simulink model "harness"  (R2024b)
settings: Solver=VariableStepAuto  StartTime=0.0  StopTime=100  FixedStep=1/100  RelTol=1e-3
InitFcn:
  | init_fn()
undefined symbols (not defined in the file): sigbuilder_block
libraries: simulink x9
settings Model: PacingRate=100  Creator=Jacopo Sini  LastModifiedBy=WxxGr
settings DataIOCC: ReturnWorkspaceOutputs=off  ReturnWorkspaceOutputsName=out1
settings OptimizationCC: ReuseModelBlockBuffer=off
settings DebuggingCC: ParameterPrecisionLossMsg=none  UnconnectedInputMsg=warning  UnconnectedOutputMsg=warning  UnconnectedLineMsg=warning
settings ModelReferenceCC: EnableRefExpFcnMdlSchedulingChecks=on  EnableParallelModelReferenceBuilds=on
settings RTWCC: GPUComputeCapability=3.5  DLArmComputeVersion=19.05
settings ConfigComp: CovMetricSettings=dcwe

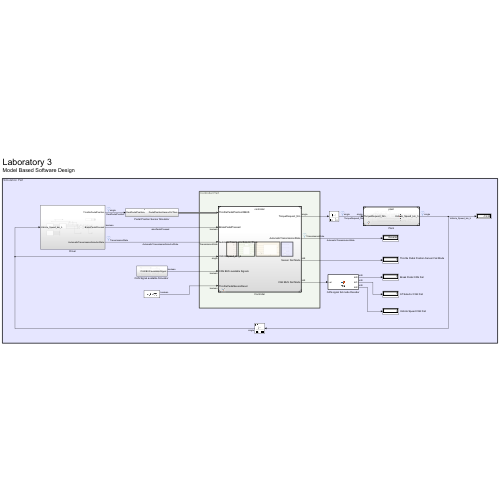
[thumbnail: Simulink's stored preview of the top-level diagram]
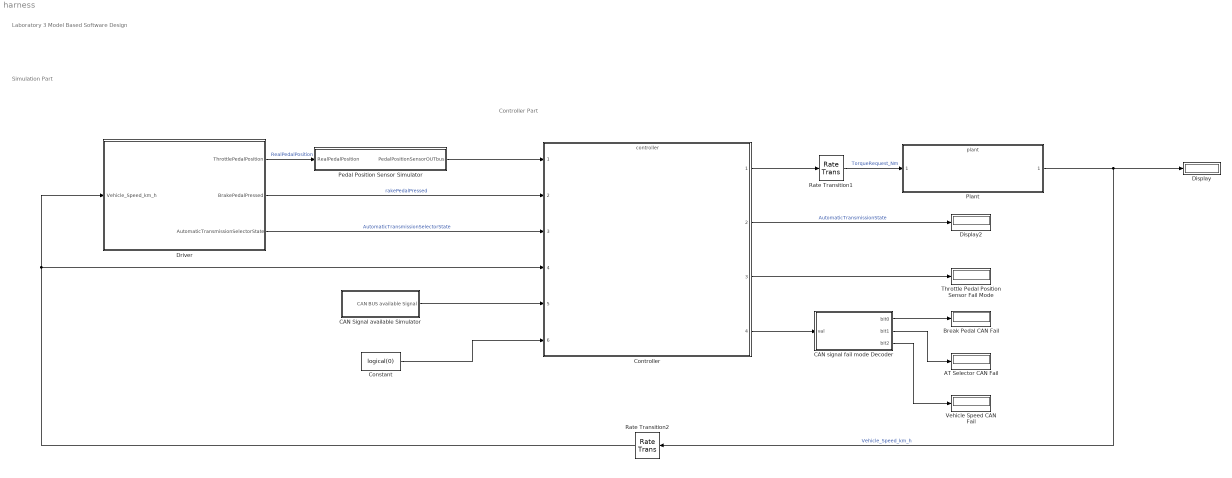
== system harness ==
  note: Simulation Part
  note: Controller Part
  note: Laboratory 3
      | Model Based Software Design
  AT Selector CAN Fail : Display
  Break Pedal CAN Fail : Display
  "CAN Signal available Simulator " : Subsystem
  CAN signal fail mode Decoder : MATLAB Function  TreatAsAtomicUnit=on
  Constant : Constant  Value=logical(0)
  Controller : ModelReference  ModelNameDialog=controller  SimulationMode=Normal  ModelReferenceVersion=7.99
  Display : Display
  Display2 : Display
  Driver : Subsystem
  Pedal Position Sensor Simulator : Subsystem
  Plant : ModelReference  ModelNameDialog=plant  SimulationMode=Normal  ModelReferenceVersion=7.4
  Rate Transition1 : RateTransition
  Rate Transition2 : RateTransition
  "Throttle Pedal Position Sensor Fail Mode " : Display
  Vehicle Speed CAN Fail : Display
  wires:
  Controller/2 -> Display2/1  "AutomaticTransmissionState"
  Controller/1 -> Rate Transition1/1
  Rate Transition2/1 -> Controller/4, Driver/1(Vehicle_Speed_km_h)
  Rate Transition1/1 -> Plant/1  "TorqueRequest_Nm"
  Plant/1 -> Rate Transition2/1, Display/1  "Vehicle_Speed_km_h"
  Driver/1(ThrottlePedalPosition) -> Pedal Position Sensor Simulator/1(RealPedalPosition)  "RealPedalPosition"
  Pedal Position Sensor Simulator/1(PedalPositionSensorOUTbus) -> Controller/1
  Controller/3 -> "Throttle Pedal Position Sensor Fail Mode "/1
  "CAN Signal available Simulator "/1(CAN BUS available Signal) -> Controller/5
  Constant/1 -> Controller/6
  Driver/3(AutomaticTransmissionSelectorState) -> Controller/3  "AutomaticTransmissionSelectorState"
  Driver/2(BrakePedalPressed) -> Controller/2  "rakePedalPressed"
  Controller/4 -> CAN signal fail mode Decoder/1(val)
  CAN signal fail mode Decoder/1(bit0) -> Break Pedal CAN Fail/1
  CAN signal fail mode Decoder/2(bit1) -> AT Selector CAN Fail/1
  CAN signal fail mode Decoder/3(bit2) -> Vehicle Speed CAN Fail/1

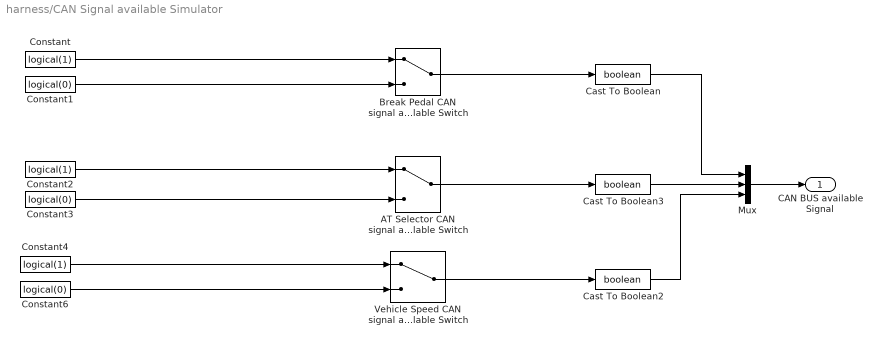
== system harness/CAN Signal available Simulator  ==
  AT Selector CAN signal available Switch : ManualSwitch
  Break Pedal CAN signal available Switch : ManualSwitch
  Cast To Boolean : DataTypeConversion  OutDataTypeStr=boolean  SaturateOnIntegerOverflow=off  RndMeth=Floor
  Cast To Boolean2 : DataTypeConversion  OutDataTypeStr=boolean  SaturateOnIntegerOverflow=off  RndMeth=Floor
  Cast To Boolean3 : DataTypeConversion  OutDataTypeStr=boolean  SaturateOnIntegerOverflow=off  RndMeth=Floor
  Constant : Constant  Value=logical(1)
  Constant1 : Constant  Value=logical(0)
  Constant2 : Constant  Value=logical(1)
  Constant3 : Constant  Value=logical(0)
  Constant4 : Constant  Value=logical(1)
  Constant6 : Constant  Value=logical(0)
  Mux : Mux  Inputs=3
  Vehicle Speed CAN signal available Switch : ManualSwitch
  CAN BUS available Signal : Outport
  wires:
  Constant/1 -> Break Pedal CAN signal available Switch/1
  Constant1/1 -> Break Pedal CAN signal available Switch/2
  Constant3/1 -> AT Selector CAN signal available Switch/2
  Constant2/1 -> AT Selector CAN signal available Switch/1
  Constant6/1 -> Vehicle Speed CAN signal available Switch/2
  Constant4/1 -> Vehicle Speed CAN signal available Switch/1
  Break Pedal CAN signal available Switch/1 -> Cast To Boolean/1
  AT Selector CAN signal available Switch/1 -> Cast To Boolean3/1
  Vehicle Speed CAN signal available Switch/1 -> Cast To Boolean2/1
  Mux/1 -> CAN BUS available Signal/1
  Cast To Boolean/1 -> Mux/1
  Cast To Boolean3/1 -> Mux/2
  Cast To Boolean2/1 -> Mux/3

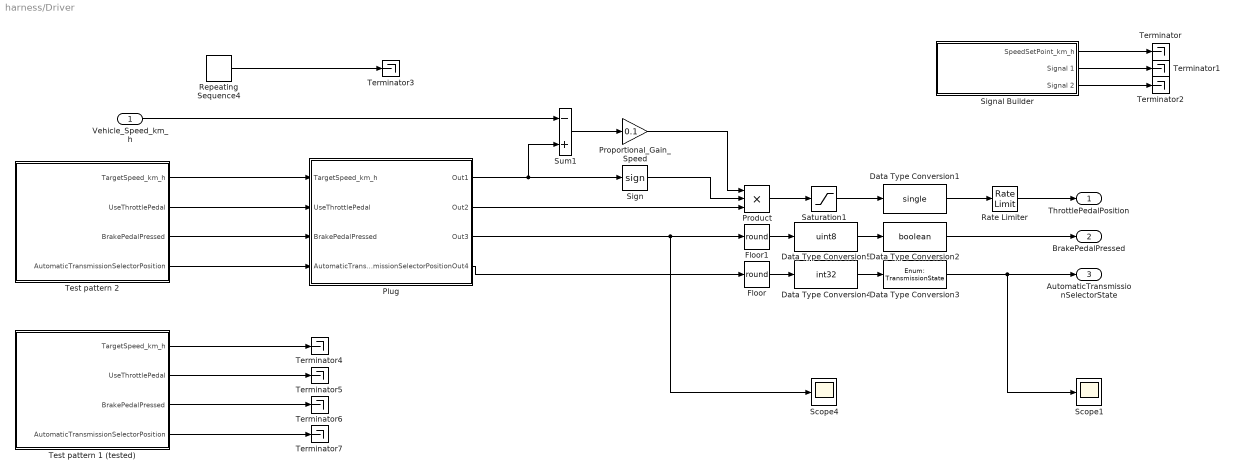
== system harness/Driver ==
  Vehicle_Speed_km_h : Inport
  Data Type Conversion1 : DataTypeConversion  OutDataTypeStr=single  SaturateOnIntegerOverflow=off  RndMeth=Floor  LockScale=on
  Data Type Conversion2 : DataTypeConversion  OutDataTypeStr=boolean  SaturateOnIntegerOverflow=off  RndMeth=Floor  LockScale=on
  Data Type Conversion3 : DataTypeConversion  OutDataTypeStr=Enum: TransmissionState  SaturateOnIntegerOverflow=off  RndMeth=Floor  LockScale=on
  Data Type Conversion4 : DataTypeConversion  OutDataTypeStr=int32  SaturateOnIntegerOverflow=off  RndMeth=Floor  LockScale=on
  Data Type Conversion5 : DataTypeConversion  OutDataTypeStr=uint8  SaturateOnIntegerOverflow=off  RndMeth=Floor  LockScale=on
  Floor : Rounding  Operator=round
  Floor1 : Rounding  Operator=round
  Plug : Subsystem
  Product : Product  Inputs=3
  Proportional_Gain_Speed : Gain  Gain=0.1
  Rate Limiter : RateLimiter  RisingSlewLimit=0.5  SampleTimeMode=inherited
  Repeating Sequence4 : simulink/Sources/Repeating Sequence  rep_seq_t=[0 10 500]  rep_seq_y=[10 0 0]
  Saturation1 : Saturate  UpperLimit=1  LowerLimit=0
  Scope1 : Scope
  Scope4 : Scope
  Sign : Signum
  Signal Builder : Subsystem  Tag=STV Subsys  LoadFcn=sigbuilder_block('load');  StartFcn=sigbuilder_block('start');  StopFcn=sigbuilder_block('stop');  ClipboardFcn=sigbuilder_block('clipboard');  mask(Sigbuilder block){tuvar=[0:10]}
      mask help: Simulink:masks:SigbuilderBlock_MD
      mask init:
      | if ~strcmp(get_param(bdroot(gcbh),'SimulationStatus'),'stopped') tuvar = sigbuilder_block('maskInit'); end
      settings: CopyFcn=sigbuilder_block('copy');  DeleteFcn=sigbuilder_block('delete');  ModelCloseFcn=sigbuilder_block('modelClose');  PreSaveFcn=sigbuilder_block('preSave');  PauseFcn=sigbuilder_block('pause');  ContinueFcn=sigbuilder_block('continue');  NameChangeFcn=sigbuilder_block('namechange');  OpenFcn=sigbuilder_block('open',[4.875 4.875 1070.25 612.375 ]);  CloseFcn=sigbuilder_block('close');
      mask Display: plot(0, 0, 100, 100,[2, 2, 32, 32, 2], [68, 8, 8, 68, 68],[32, 2], [38, 38], [32, 19, 2],[53, 60, 44], [32, 17, 17, 2],[16, 16, 31, 31]);txt = getActiveGroup(gcbh);text(2, 100, txt,'verticalAlignment', 'top');
  Sum1 : Sum  Inputs=-+
  Terminator{,1..7} (8 alike) : Terminator
  Test pattern 1 (tested) : Subsystem
  Test pattern 2 : Subsystem
  ThrottlePedalPosition : Outport
  BrakePedalPressed : Outport  Port=2
  AutomaticTransmissionSelectorState : Outport  Port=3  OutDataTypeStr=Enum: TransmissionState
  wires:
  Data Type Conversion1/1 -> Rate Limiter/1
  Data Type Conversion5/1 -> Data Type Conversion2/1
  Data Type Conversion3/1 -> Scope1/1, AutomaticTransmissionSelectorState/1
  Floor/1 -> Data Type Conversion4/1
  Data Type Conversion4/1 -> Data Type Conversion3/1
  Floor1/1 -> Data Type Conversion5/1
  Product/1 -> Saturation1/1
  Sum1/1 -> Proportional_Gain_Speed/1
  Sign/1 -> Product/2
  Saturation1/1 -> Data Type Conversion1/1
  Rate Limiter/1 -> ThrottlePedalPosition/1
  Repeating Sequence4/1 -> Terminator3/1
  Vehicle_Speed_km_h/1 -> Sum1/1
  Proportional_Gain_Speed/1 -> Product/1
  Plug/1(Out1) -> Sum1/2, Sign/1
  Plug/3(Out3) -> Scope4/1, Floor1/1
  Plug/4(Out4) -> Floor/1
  Plug/2(Out2) -> Product/3
  Test pattern 2/1(TargetSpeed_km_h) -> Plug/1(TargetSpeed_km_h)
  Test pattern 2/2(UseThrottlePedal) -> Plug/2(UseThrottlePedal)
  Test pattern 2/3(BrakePedalPressed) -> Plug/3(BrakePedalPressed)
  Test pattern 2/4(AutomaticTransmissionSelectorPosition) -> Plug/4(AutomaticTransmissionSelectorPosition)
  Data Type Conversion2/1 -> BrakePedalPressed/1
  Signal Builder/1(SpeedSetPoint_km_h) -> Terminator/1
  Signal Builder/2(Signal 1) -> Terminator1/1
  Signal Builder/3(Signal 2) -> Terminator2/1
  Test pattern 1 (tested)/4(AutomaticTransmissionSelectorPosition) -> Terminator7/1
  Test pattern 1 (tested)/3(BrakePedalPressed) -> Terminator6/1
  Test pattern 1 (tested)/2(UseThrottlePedal) -> Terminator5/1
  Test pattern 1 (tested)/1(TargetSpeed_km_h) -> Terminator4/1

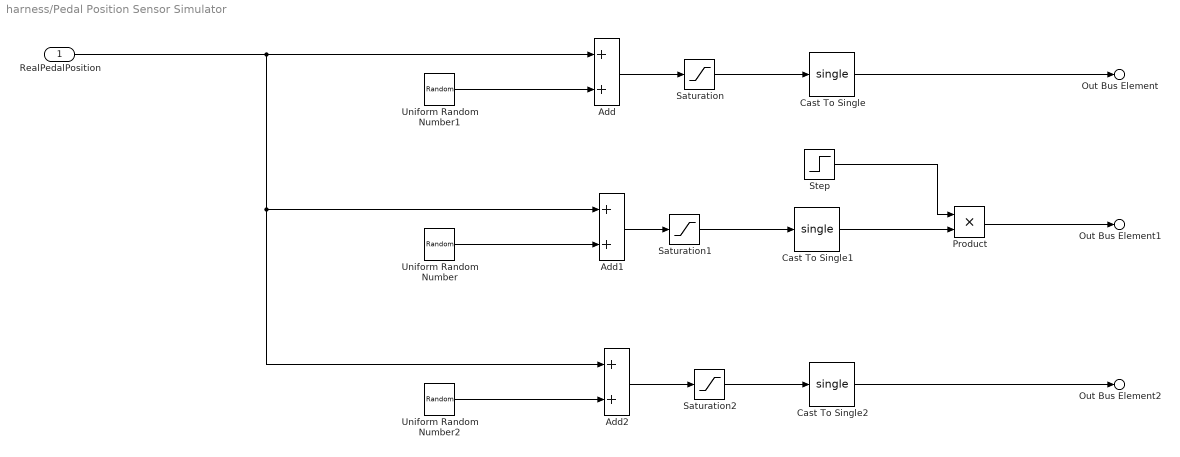
== system harness/Pedal Position Sensor Simulator ==
  RealPedalPosition : Inport
  Add : Sum
  Add1 : Sum
  Add2 : Sum
  Cast To Single : DataTypeConversion  OutDataTypeStr=single  SaturateOnIntegerOverflow=off  RndMeth=Floor
  Cast To Single1 : DataTypeConversion  OutDataTypeStr=single  SaturateOnIntegerOverflow=off  RndMeth=Floor
  Cast To Single2 : DataTypeConversion  OutDataTypeStr=single  SaturateOnIntegerOverflow=off  RndMeth=Floor
  Product : Product
  Saturation : Saturate  UpperLimit=1  LowerLimit=0
  Saturation1 : Saturate  UpperLimit=1  LowerLimit=0
  Saturation2 : Saturate  UpperLimit=1  LowerLimit=0
  Step : Step  Time=10  Before=1  OutDataTypeStr=single  SampleTime=0
  Uniform Random Number : UniformRandomNumber  Minimum=-0.0005  Maximum=0.0005  Seed=randi(99999)  SampleTime=0.001
  Uniform Random Number1 : UniformRandomNumber  Minimum=-0.0005  Maximum=0.0005  Seed=randi(99999)  SampleTime=0.001
  Uniform Random Number2 : UniformRandomNumber  Minimum=-0.0005  Maximum=0.0005  Seed=randi(99999)  SampleTime=0.001
  Out Bus Element : Outport  PortName=PedalPositionSensorOUTbus  Element=PedalPositionSensor1OUT
  Out Bus Element1 : Outport  PortName=PedalPositionSensorOUTbus  Element=PedalPositionSensor2OUT
  Out Bus Element2 : Outport  PortName=PedalPositionSensorOUTbus  Element=PedalPositionSensor3OUT
  wires:
  Add/1 -> Saturation/1
  Saturation/1 -> Cast To Single/1
  Uniform Random Number1/1 -> Add/2
  Add1/1 -> Saturation1/1
  Saturation1/1 -> Cast To Single1/1
  Uniform Random Number2/1 -> Add2/2
  Saturation2/1 -> Cast To Single2/1
  Cast To Single2/1 -> Out Bus Element2/1
  Add2/1 -> Saturation2/1
  RealPedalPosition/1 -> Add2/1, Add1/1, Add/1
  Uniform Random Number/1 -> Add1/2
  Cast To Single/1 -> Out Bus Element/1
  Cast To Single1/1 -> Product/2
  Step/1 -> Product/1
  Product/1 -> Out Bus Element1/1

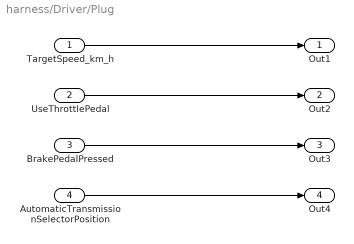
== system harness/Driver/Plug ==
  TargetSpeed_km_h : Inport
  UseThrottlePedal : Inport  Port=2
  BrakePedalPressed : Inport  Port=3
  AutomaticTransmissionSelectorPosition : Inport  Port=4
  Out1 : Outport
  Out2 : Outport  Port=2
  Out3 : Outport  Port=3
  Out4 : Outport  Port=4
  wires:
  TargetSpeed_km_h/1 -> Out1/1
  UseThrottlePedal/1 -> Out2/1
  BrakePedalPressed/1 -> Out3/1
  AutomaticTransmissionSelectorPosition/1 -> Out4/1

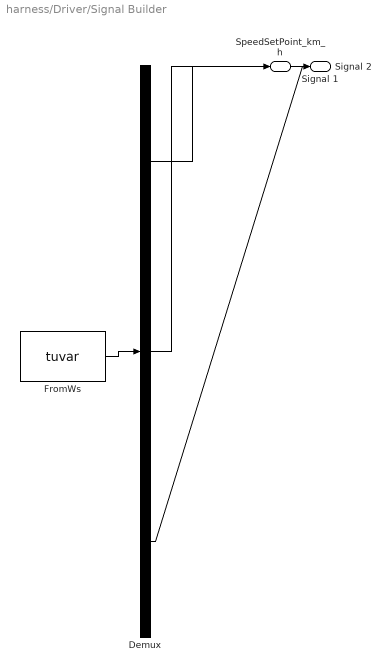
== system harness/Driver/Signal Builder ==
  Demux : Demux  Tag=STV Demux  Outputs=3
      settings: DisplayOption=none
  FromWs : FromWorkspace  Tag=STV FromWs  VariableName=tuvar
      SigBuilderData=|
      | common.afterFinalStr = 'Extrapolate'
      | common.sampleTime = 0
      | dataSet.timeRange = [0 500]
      | dataSet.name = 'Group 1'
      | sbobj.Groups.Name = 'Group 1'
      | sbobj.Groups.Signals(1).Name = 'SpeedSetPoint_km_h'
      | sbobj.Groups.Signals(1).XData = [0 2.165 2.165 6 6 500]
      | sbobj.Groups.Signals(1).YData = [0 0 1 1 0.53 0]
      | sbobj.Groups.Signals(2).Name = 'Signal 1'
      | sbobj.Groups.Signals(2).XData = [0 0.5 0.5 1 1 1.5 1.5 2 2 2.5 2.5 3 ... (2000 elements, 1x2000)]
      | sbobj.Groups.Signals(2).YData = [2 2 0 0 2 2 0 0 2 2 0 0 ... (2000 elements, 1x2000)]
      | sbobj.Groups.Signals(3).Name = 'Signal 2'
      | sbobj.Groups.Signals(3).XData = [0 63.5 63.5 500]
      | sbobj.Groups.Signals(3).YData = [0 0 1 1]
      | sbobj.Groups.TimeRange = [0 500]
  SpeedSetPoint_km_h : Outport  Tag=STV Outport
  Signal 1 : Outport  Tag=STV Outport  Port=2
  Signal 2 : Outport  Tag=STV Outport  Port=3
  wires:
  Demux/1 -> SpeedSetPoint_km_h/1
  FromWs/1 -> Demux/1
  Demux/2 -> Signal 1/1
  Demux/3 -> Signal 2/1

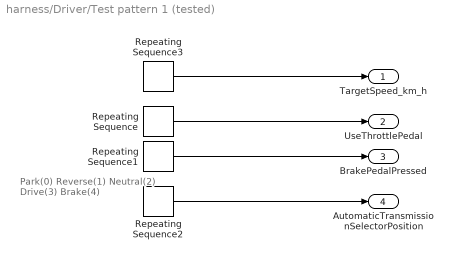
== system harness/Driver/Test pattern 1 (tested) ==
  note: Park(0)
      | Reverse(1)
      | Neutral(2)
      | Drive(3)
      | Brake(4)
  Repeating Sequence : simulink/Sources/Repeating Sequence  rep_seq_t=[0 3.9 4 500]  rep_seq_y=[0 0 1 1]
  Repeating Sequence1 : simulink/Sources/Repeating Sequence  rep_seq_t=[0 2.999 3 49.9 50.0 52.0 52.1 500]  rep_seq_y=[1 1 0 0 1 1 0 0]
  Repeating Sequence2 : simulink/Sources/Repeating Sequence  rep_seq_t=[0 1.999 2 10 49.9 50.0 500]  rep_seq_y=[0 0 4 4 4 1 1]
  Repeating Sequence3 : simulink/Sources/Repeating Sequence  rep_seq_t=[0 3.9 4 29.9 30 39.9 40 52.9 53 500]  rep_seq_y=[0 0 90 90 60 60 0 0 -20 -20]
  TargetSpeed_km_h : Outport
  UseThrottlePedal : Outport  Port=2
  BrakePedalPressed : Outport  Port=3
  AutomaticTransmissionSelectorPosition : Outport  Port=4
  wires:
  Repeating Sequence2/1 -> AutomaticTransmissionSelectorPosition/1
  Repeating Sequence/1 -> UseThrottlePedal/1
  Repeating Sequence1/1 -> BrakePedalPressed/1
  Repeating Sequence3/1 -> TargetSpeed_km_h/1

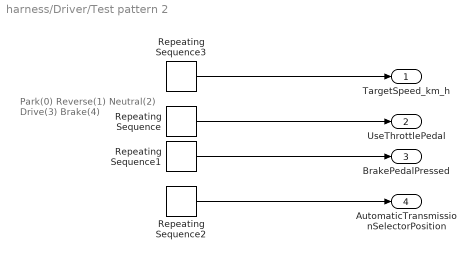
== system harness/Driver/Test pattern 2 ==
  note: Park(0)
      | Reverse(1)
      | Neutral(2)
      | Drive(3)
      | Brake(4)
  Repeating Sequence : simulink/Sources/Repeating Sequence  rep_seq_t=[0 3.9 4 500]  rep_seq_y=[0 0 1 1]
  Repeating Sequence1 : simulink/Sources/Repeating Sequence  rep_seq_t=[0 2.999 3 49.9 80.0 82.0 92.1 500]  rep_seq_y=[1 1 0 0 1 1 0 0]
  Repeating Sequence2 : simulink/Sources/Repeating Sequence  rep_seq_t=[0 1.999 2 10 79.9 80.0 500]  rep_seq_y=[0 0 4 4 4 1 1]
  Repeating Sequence3 : simulink/Sources/Repeating Sequence  rep_seq_t=[0 3.9 4 29.9 30 39.9 40 82.9 83 500]  rep_seq_y=[0 0 90 90 60 60 0 0 -20 -20]
  TargetSpeed_km_h : Outport
  UseThrottlePedal : Outport  Port=2
  BrakePedalPressed : Outport  Port=3
  AutomaticTransmissionSelectorPosition : Outport  Port=4
  wires:
  Repeating Sequence2/1 -> AutomaticTransmissionSelectorPosition/1
  Repeating Sequence/1 -> UseThrottlePedal/1
  Repeating Sequence1/1 -> BrakePedalPressed/1
  Repeating Sequence3/1 -> TargetSpeed_km_h/1

== matlab function harness/CAN signal fail mode Decoder ==
  data: val input; bit0 output; bit1 output; bit2 output
function [bit0,bit1,bit2]= fcn(val)

    bit0 = bitand(val, 1);
    bit1 = bitand(bitshift(val, -1), 1);
    bit2 = bitand(bitshift(val, -2), 1);

end
